simulink model "MOD5Counter"  (R2020b)
settings: Solver=VariableStepAuto  StartTime=0.0  StopTime=10.0  RelTol=1e-3
settings Model: EnablePacing=on  PacingRate=0.180000  Creator=vijay jagtap  LastModifiedBy=vijay jagtap

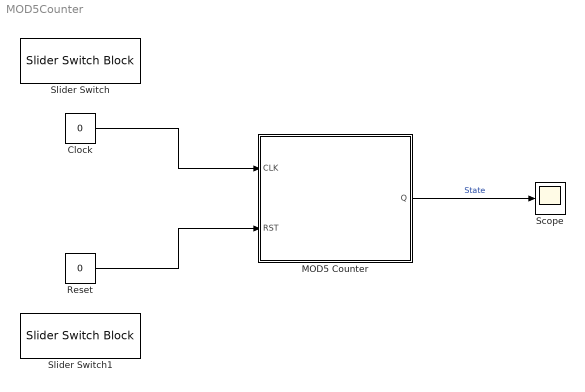
== system MOD5Counter ==
  Clock : Constant  Value=0
  MOD5 Counter : Stateflow chart  TreatAsAtomicUnit=on
  Reset : Constant  Value=0
  Scope : Scope
  Slider Switch : SliderSwitchBlock
      settings: Values={{'Off', 'On'}, [0 1]}
  Slider Switch1 : SliderSwitchBlock
      settings: Values={{'Off', 'On'}, [0 1]}
  wires:
  MOD5 Counter/1(Q) -> Scope/1  "State"
  Clock/1 -> MOD5 Counter/1(CLK)
  Reset/1 -> MOD5 Counter/2(RST)

== stateflow chart MOD5Counter/MOD5 Counter ==
  state Clock
  state Reset
    Q = 0;
  state MOD_5
    state Reset_Control [parallel]
      settings: executionOrder=1
      state IDLE
      state Up
      state Reset_State
      (default) -> IDLE
      IDLE -> Reset_State [order 2] : [Q ==4]
          | /{send(Reset,States)}
      IDLE -> Up [order 1] : [Q ~= 4]
          | /{send(UP,States)}
      Up -> IDLE : after(1,msec)
      Reset_State -> IDLE : after(1,msec)
    state States [parallel]
      settings: executionOrder=2
      state state_0
        entry:
        Q = 0;
      state state_1
        entry:
        Q = 1;
      state state_2
        entry:
        Q = 2;
      state state_3
        entry:
        Q = 3;
      state state_4
        entry:
        Q = 4;
      state_4 -> state_0 : Reset
      (default) -> state_0
      state_0 -> state_1 : UP
      state_1 -> state_2 : UP
      state_2 -> state_3 : UP
      state_3 -> state_4 : UP
  (default) -> Clock
  Clock -> MOD_5 : [CLK == 1]
  MOD_5 -> Clock [order 1] : [CLK == 0]
  Reset -> MOD_5 : [RST == 0]
  MOD_5 -> Reset [order 2] : [RST == 1]
  data: CLK input; Q output; RST input
  events: UP local FUNCTION_CALL_EVENT; Reset local FUNCTION_CALL_EVENT
